simulink model "PruebaAdc"  (R2016b)
settings: Solver=FixedStepDiscrete  StartTime=0.0  StopTime=inf  FixedStep=0.01  RelTol=1e-3  EnableMultiTasking=on
libraries: arduinolib x8, simulink x7, simulink_extras x1
settings Model: SimulationMode=external  ExtModeTrigDuration=2  Creator=Julian  LastModifiedBy=Julian
settings OptimizationCC: MaxStackSize=64
settings DebuggingCC: ParameterTunabilityLossMsg=error
settings HardwareCC: ProdBitPerInt=16  ProdBitPerPointer=16  ProdBitPerSizeT=16  ProdBitPerPtrDiffT=16  ProdLargestAtomicFloat=None  ProdWordSize=8  ProdHWDeviceType=Atmel->AVR
settings RTWCC: SystemTargetFile=ert.tlc  HardwareBoard=Arduino Mega 2560  TLCOptions=-aInlineSetEventsForThisBaseRateFcn=TLC_FALSE -aSuppressMultiTaskScheduler=TLC_FALSE -aRateBasedStepFcn=1  TemplateMakefile=ert_default_tmf  Description=Embedded Coder  GenerateReport=on  Toolchain=Arduino AVR  BuildConfiguration=Faster Runs  IncludeHyperlinkInReport=on  LaunchReport=on  GenerateTraceInfo=on  GenerateTraceReport=on  GenerateTraceReportSl=on  GenerateTraceReportSf=on  GenerateTraceReportEml=on
settings CodeAppCC: ForceParamTrailComments=on  IgnoreCustomStorageClasses=off  OperatorAnnotations=on  SimulinkDataObjDesc=on  SFDataObjDesc=on  MATLABFcnDesc=on  InsertBlockDesc=on  MATLABSourceComments=on
settings ERTTargetCC: SupportContinuousTime=on  SupportVariableSizeSignals=on

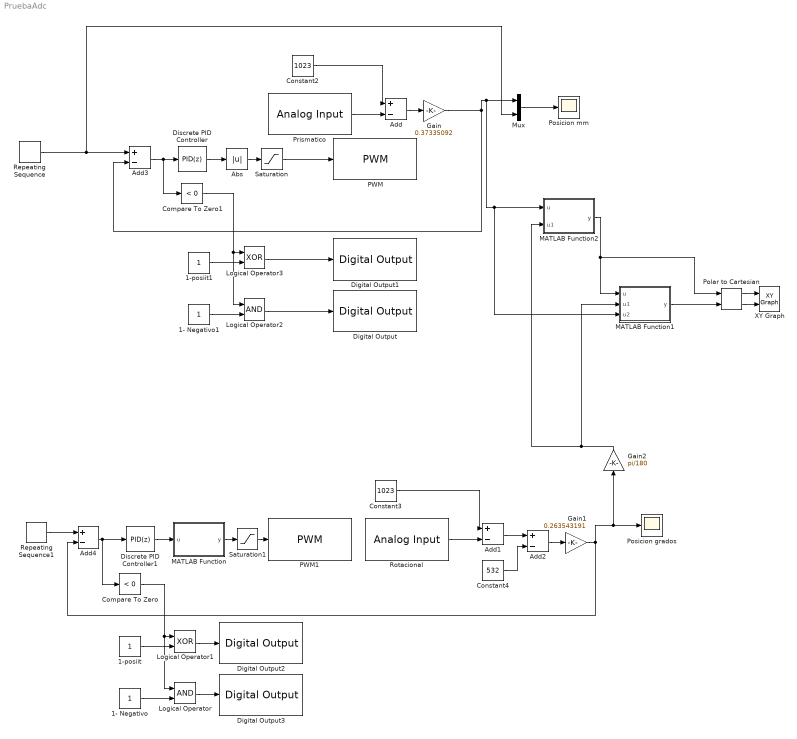
== system PruebaAdc ==
  1- Negativo : Constant
  1- Negativo1 : Constant
  1-posiit : Constant
  1-posiit1 : Constant
  Abs : Abs
  Add{,1..4} (5 alike) : Sum  Inputs=+-
  Compare To Zero : simulink/Logic and Bit Operations/Compare To Zero  relop=<  OutDataTypeStr=boolean
  Compare To Zero1 : simulink/Logic and Bit Operations/Compare To Zero  relop=<  OutDataTypeStr=boolean
  Constant2 : Constant  Value=1023
  Constant3 : Constant  Value=1023
  Constant4 : Constant  Value=532
  Digital Output : arduinolib/Digital Output  pinNumber=2  blockPlatform=arduino
  Digital Output1 : arduinolib/Digital Output  pinNumber=3  blockPlatform=arduino
  Digital Output2 : arduinolib/Digital Output  pinNumber=7  blockPlatform=arduino
  Digital Output3 : arduinolib/Digital Output  pinNumber=6  blockPlatform=arduino
  Discrete PID Controller : simulink/Continuous/PID Controller  Controller=PID  TimeDomain=Discrete-time  SampleTime=-1  IntegratorMethod=Forward Euler  FilterMethod=Forward Euler  Form=Parallel  UseFilter=on  ControllerParametersSource=internal  P=270  I=0  D=0  N=100  InitialConditionSource=internal  InitialConditionForIntegrator=0  InitialConditionForFilter=0  ExternalReset=none  LimitOutput=off  UpperSaturationLimit=inf  LowerSaturationLimit=-inf  LinearizeAsGain=off  AntiWindupMode=none  Kb=1  TrackingMode=off  Kt=1  PParamMin=[]  PParamMax=[]  IParamMin=[]  IParamMax=[]  DParamMin=[]  DParamMax=[]  NParamMin=[]  NParamMax=[]  KbParamMin=[]  KbParamMax=[]  KtParamMin=[]  KtParamMax=[]  POutMin=[]  POutMax=[]  IOutMin=[]  IOutMax=[]  DOutMin=[]  DOutMax=[]  NOutMin=[]  NOutMax=[]  KbOutMin=[]  KbOutMax=[]  KtOutMin=[]  KtOutMax=[]  IntegratorOutMin=[]  IntegratorOutMax=[]  FilterOutMin=[]  FilterOutMax=[]  SumOutMin=[]  SumOutMax=[]  SumI1OutMin=[]  SumI1OutMax=[]  SumI2OutMin=[]  SumI2OutMax=[]  SumI3OutMin=[]  SumI3OutMax=[]  SumDOutMin=[]  SumDOutMax=[]  SaturationOutMin=[]  SaturationOutMax=[]  IntegratorContinuousStateAttributes=''  IntegratorStateMustResolveToSignalObject=off  IntegratorRTWStateStorageClass=Auto  FilterContinuousStateAttributes=''  FilterStateMustResolveToSignalObject=off  FilterRTWStateStorageClass=Auto  DifferentiatorICPrevScaledInput=0  DifferentiatorOutMin=[]  DifferentiatorOutMax=[]
  Discrete PID Controller1 : simulink/Continuous/PID Controller  Controller=PID  TimeDomain=Discrete-time  SampleTime=-1  IntegratorMethod=Forward Euler  FilterMethod=Forward Euler  Form=Parallel  UseFilter=on  ControllerParametersSource=internal  P=10  I=1.5  D=0.1  N=100  InitialConditionSource=internal  InitialConditionForIntegrator=0  InitialConditionForFilter=0  ExternalReset=none  LimitOutput=off  UpperSaturationLimit=inf  LowerSaturationLimit=-inf  LinearizeAsGain=off  AntiWindupMode=none  Kb=1  TrackingMode=off  Kt=1  PParamMin=[]  PParamMax=[]  IParamMin=[]  IParamMax=[]  DParamMin=[]  DParamMax=[]  NParamMin=[]  NParamMax=[]  KbParamMin=[]  KbParamMax=[]  KtParamMin=[]  KtParamMax=[]  POutMin=[]  POutMax=[]  IOutMin=[]  IOutMax=[]  DOutMin=[]  DOutMax=[]  NOutMin=[]  NOutMax=[]  KbOutMin=[]  KbOutMax=[]  KtOutMin=[]  KtOutMax=[]  IntegratorOutMin=[]  IntegratorOutMax=[]  FilterOutMin=[]  FilterOutMax=[]  SumOutMin=[]  SumOutMax=[]  SumI1OutMin=[]  SumI1OutMax=[]  SumI2OutMin=[]  SumI2OutMax=[]  SumI3OutMin=[]  SumI3OutMax=[]  SumDOutMin=[]  SumDOutMax=[]  SaturationOutMin=[]  SaturationOutMax=[]  IntegratorContinuousStateAttributes=''  IntegratorStateMustResolveToSignalObject=off  IntegratorRTWStateStorageClass=Auto  FilterContinuousStateAttributes=''  FilterStateMustResolveToSignalObject=off  FilterRTWStateStorageClass=Auto  DifferentiatorICPrevScaledInput=0  DifferentiatorOutMin=[]  DifferentiatorOutMax=[]
  Gain : Gain  Gain=0.37335092
  Gain1 : Gain  Gain=0.263543191
  Gain2 : Gain  Gain=pi/180
  Logical Operator : Logic  AllPortsSameDT=off  OutDataTypeStr=boolean
  Logical Operator1 : Logic  Operator=XOR  AllPortsSameDT=off  OutDataTypeStr=boolean
  Logical Operator2 : Logic  AllPortsSameDT=off  OutDataTypeStr=boolean
  Logical Operator3 : Logic  Operator=XOR  AllPortsSameDT=off  OutDataTypeStr=boolean
  MATLAB Function : MATLAB Function  TreatAsAtomicUnit=on
  MATLAB Function1 : MATLAB Function  TreatAsAtomicUnit=on
  MATLAB Function2 : MATLAB Function  TreatAsAtomicUnit=on
  Mux : Mux  Inputs=2
  PWM : arduinolib/PWM  pinNumber=4  blockPlatform=arduino
  PWM1 : arduinolib/PWM  pinNumber=5  blockPlatform=arduino
  Polar to Cartesian : simulink_extras/Transformations/Polar to Cartesian
  Posicion grados : Scope
  Posicion mm : Scope
  Prismatico : arduinolib/Analog Input  pinNumber=0  sampleTime=0.01  blockPlatform=arduino
  Repeating Sequence : simulink/Sources/Repeating Sequence  rep_seq_t=t  rep_seq_y=d
  Repeating Sequence1 : simulink/Sources/Repeating Sequence  rep_seq_t=t  rep_seq_y=phi
  Rotacional : arduinolib/Analog Input  pinNumber=1  sampleTime=0.01  blockPlatform=arduino
  Saturation : Saturate  UpperLimit=255  LowerLimit=0
  Saturation1 : Saturate  UpperLimit=255  LowerLimit=0
  XY Graph : simulink/Sinks/XY Graph  xmin=-200  xmax=200  ymin=-200  ymax=200  st=-1
  wires:
  Prismatico/1 -> Add/2
  Constant2/1 -> Add/1
  Add/1 -> Gain/1
  Gain/1 -> MATLAB Function1/3(u2), MATLAB Function2/1(u), Mux/1, Add3/2
  Discrete PID Controller/1 -> Abs/1
  Rotacional/1 -> Add1/2
  Constant3/1 -> Add1/1
  Add2/1 -> Gain1/1
  Add1/1 -> Add2/1
  Constant4/1 -> Add2/2
  Repeating Sequence1/1 -> Add4/1
  Add4/1 -> Discrete PID Controller1/1, Compare To Zero/1
  1-posiit/1 -> Logical Operator1/2
  Compare To Zero/1 -> Logical Operator1/1, Logical Operator/1
  Logical Operator1/1 -> Digital Output2/1
  1- Negativo/1 -> Logical Operator/2
  Logical Operator/1 -> Digital Output3/1
  Discrete PID Controller1/1 -> MATLAB Function/1(u)
  Add3/1 -> Compare To Zero1/1, Discrete PID Controller/1
  1-posiit1/1 -> Logical Operator3/2
  Compare To Zero1/1 -> Logical Operator3/1, Logical Operator2/1
  Logical Operator3/1 -> Digital Output1/1
  1- Negativo1/1 -> Logical Operator2/2
  Logical Operator2/1 -> Digital Output/1
  Repeating Sequence/1 -> Mux/2, Add3/1
  Saturation/1 -> PWM/1
  Abs/1 -> Saturation/1
  MATLAB Function/1(y) -> Saturation1/1
  Saturation1/1 -> PWM1/1
  Mux/1 -> Posicion mm/1
  Gain1/1 -> Gain2/1, Posicion grados/1, Add4/2
  Gain2/1 -> MATLAB Function1/2(u1), MATLAB Function2/2(u1)
  MATLAB Function2/1(y) -> Polar to Cartesian/1, MATLAB Function1/1(u)
  MATLAB Function1/1(y) -> Polar to Cartesian/2
  Polar to Cartesian/1 -> XY Graph/1
  Polar to Cartesian/2 -> XY Graph/2

== matlab function PruebaAdc/MATLAB Function1 ==
  data: u input; y output; u1 input; u2 input
function y = fcn(u,u1,u2)
if u2<146
d=-sqrt(u^2-(180*sin(u1))^2);
else
d=sqrt(u^2-(180*sin(u1))^2);
end
y = atan2(180*sin(u1),d);

== matlab function PruebaAdc/MATLAB Function ==
  data: u input; y output
function y = fcn(u)
if u>0
    y=2.3*u;
else
    y =-1*u;
end
end

== matlab function PruebaAdc/MATLAB Function2 ==
  data: u input; y output; u1 input
function y = fcn(u,u1)

y = sqrt(((300-u)^2)+32400-(2*(300-u)*180*cos(u1)));
